simulink model "CascadFilter"  (R2020b)
settings: Solver=VariableStepAuto  StartTime=0.0  StopTime=10.0  RelTol=1e-3
settings Model: Creator=BIDITA PAUL  LastModifiedBy=BIDITA PAUL
settings DataIOCC: SaveOutput=off  SaveTime=off

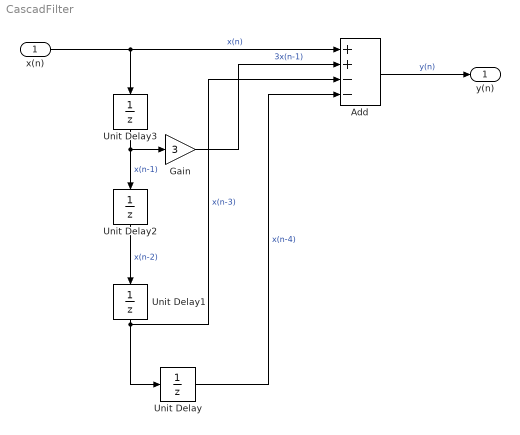
== system CascadFilter ==
  x(n) : Inport  OutDataTypeStr=double  PortDimensions=1  SampleTime=[0,1]
  Add : Sum  Inputs=++--
  Gain : Gain  Gain=3
  Unit Delay{,1..3} (4 alike) : UnitDelay  SampleTime=-1  HasFrameUpgradeWarning=on
  y(n) : Outport  OutDataTypeStr=double  PortDimensions=1  SampleTime=[0,1]
  wires:
  Unit Delay3/1 -> Unit Delay2/1, Gain/1  "x(n-1)"
  Unit Delay2/1 -> Unit Delay1/1  "x(n-2)"
  Add/1 -> y(n)/1  "y(n)"
  Unit Delay1/1 -> Unit Delay/1, Add/3  "x(n-3)"
  Unit Delay/1 -> Add/4  "x(n-4)"
  Gain/1 -> Add/2  "3x(n-1)"
  x(n)/1 -> Unit Delay3/1, Add/1  "x(n)"
